simulink model "Demo_Shore"  (R2014a)
settings: Solver=FixedStepDiscrete  SolverMode=SingleTasking  StartTime=0.0  StopTime=inf  FixedStep=0.01  RelTol=1e-3
PostLoadFcn:
  | h_RPStest = RPStest;
model workspace (MAT data in the model file):
  gtest = 0
undefined symbols (not defined in the file or in its folder): avert, avert_gaze_dirs_chance, avert_gaze_duration_factor, avert_head_frequency_factor, avert_head_speed, BML, BML1, BML2, bmlsL, bmlsM, bodyBusyFlag, clock, emotion_amount_factor, faceBusyFlag, fileID, GAZE_WIN, gazing, mutual_gaze_duration_factor, P, pose_chanc_factor, pose_chance_factor, pose_change_flag, pose_frequency_factor, pose_lean, pose_lean_flag, pose_selfAdaptor_chance_factor, pose_speed, pr, serial, STATE_BEFORE, STATE_GO, STATE_OVER, STATE_READY, Stateflow
libraries: simulink x23, instrumentlib x6, lib_affectiveChar_behavior x3, realtime_pacer_lib x2, lib_affectiveChar_input x1
(part 2 of 7)

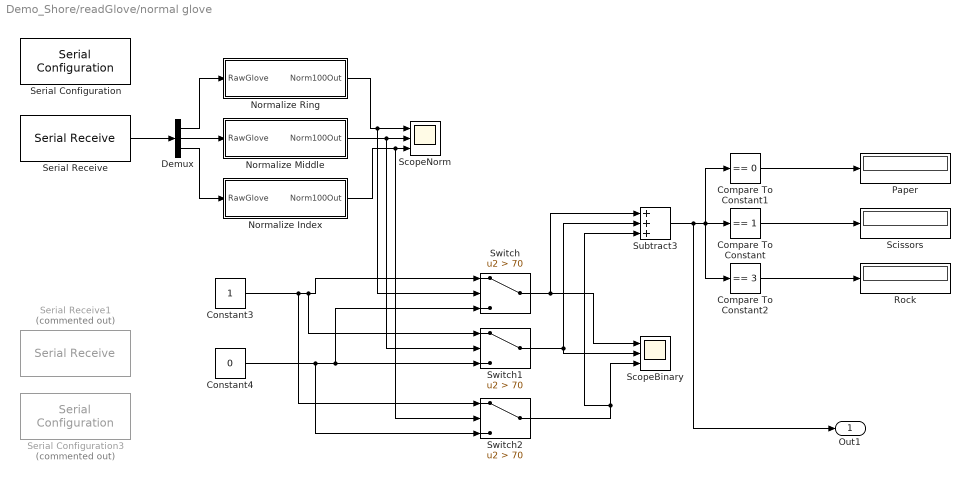
== system Demo_Shore/readGlove/normal glove ==
  Compare To Constant : simulink/Logic and Bit Operations/Compare To Constant  relop===  const=1  OutDataTypeStr=boolean
  Compare To Constant1 : simulink/Logic and Bit Operations/Compare To Constant  relop===  const=0  OutDataTypeStr=boolean
  Compare To Constant2 : simulink/Logic and Bit Operations/Compare To Constant  relop===  const=3  OutDataTypeStr=boolean
  Constant3 : Constant
  Constant4 : Constant  Value=0
  Demux : Demux  Outputs=3
  Normalize Index : Subsystem
  Normalize Middle : Subsystem
  Normalize Ring : Subsystem
  Paper : Display
  Rock : Display
  Scissors : Display
  ScopeBinary : Scope  NumInputPorts=3
      settings: YMin=-0.5~-0.5~-0.5  YMax=1.5~1.5~1.5
  ScopeNorm : Scope  NumInputPorts=3
      settings: TimeRange=10  YMin=-20~-20~-20  YMax=150~150~150
  Serial Configuration : instrumentlib/Serial Configuration  Priority=-200000  ComPortMenu=COM4  ComPort=COM4  ObjConstructor=serial('COM4');  BaudRate=9600  DataBits=8  Parity=none  StopBits=1  FlowControl=none  Timeout=10  ByteOrder=LittleEndian
  Serial Configuration3 : instrumentlib/Serial Configuration  Priority=-200000  Commented=on  ComPortMenu=<Please select a port...>  ComPort=COM5  ObjConstructor=serial('COM5');  BaudRate=9600  DataBits=8  Parity=none  StopBits=1  FlowControl=none  Timeout=10  ByteOrder=LittleEndian
  Serial Receive : instrumentlib/Serial Receive  ComPortMenu=COM4  ComPort=COM4  ObjConstructor=serial('COM4');  Terminator=<none>  DataSize="[3  1]"  DataType=uint8  EnableBlockingMode=on  ActionDataUnavailable=Output last received value  CustomValue=0  SampleTime=0.01
  Serial Receive1 : instrumentlib/Serial Receive  Commented=on  ComPortMenu=<Please select a port...>  ComPort=COM5  ObjConstructor=serial('COM5');  Terminator=<none>  DataSize="[3  1]"  DataType=uint8  EnableBlockingMode=on  ActionDataUnavailable=Output last received value  CustomValue=0  SampleTime=0.01
  Subtract3 : Sum  Inputs=+++
  Switch : Switch  Criteria=u2 > Threshold  Threshold=70
  Switch1 : Switch  Criteria=u2 > Threshold  Threshold=70
  Switch2 : Switch  Criteria=u2 > Threshold  Threshold=70
  Out1 : Outport
  wires:
  Demux/1 -> Normalize Ring/1(RawGlove)
  Demux/2 -> Normalize Middle/1(RawGlove)
  Demux/3 -> Normalize Index/1(RawGlove)
  Switch/1 -> ScopeBinary/1, Subtract3/1
  Constant3/1 -> Switch2/1, Switch1/1, Switch/1
  Constant4/1 -> Switch2/3, Switch1/3, Switch/3
  Switch1/1 -> ScopeBinary/2, Subtract3/2
  Switch2/1 -> Subtract3/3, ScopeBinary/3
  Subtract3/1 -> Compare To Constant/1, Compare To Constant2/1, Compare To Constant1/1, Out1/1
  Compare To Constant1/1 -> Paper/1
  Compare To Constant/1 -> Scissors/1
  Compare To Constant2/1 -> Rock/1
  Normalize Index/1(Norm100Out) -> Switch2/2, ScopeNorm/3
  Normalize Ring/1(Norm100Out) -> Switch/2, ScopeNorm/1
  Normalize Middle/1(Norm100Out) -> ScopeNorm/2, Switch1/2
  Serial Receive/1 -> Demux/1

== system Demo_Shore/readSHORE/smile ==
  In1 : Inport
  ifSmile : MATLAB Function  TreatAsAtomicUnit=on
  Out1 : Outport
  wires:
  ifSmile/1(y) -> Out1/1
  In1/1 -> ifSmile/1(u)

== system Demo_Shore/GazeFollowSubsystem/reactiveGaze/createGazePawn/sendBML ==
  In1 : Inport  OutDataTypeStr=double  PortDimensions=[1000 1]
  f : TriggerPort  TriggerType=function-call
      settings: CopyFcn=Stateflow.SLINSF.SimulinkMan.removeBlockPreDeleteFcn  PreDeleteFcn=Stateflow.SLINSF.SimulinkMan.unsafePredeleteFcn
  C++ S-Function2 : S-Function  FunctionName=yarpSendText_sfun  Parameters='/sim/out/bml8', '/SB/in/bml'  EnableBusSupport=off
  wires:
  In1/1 -> C++ S-Function2/1

== system Demo_Shore/GazeFollowSubsystem/reactiveGaze/createGazePawn/sendSBM ==
  In2 : Inport  OutDataTypeStr=double  PortDimensions=[1000 1]
  f : TriggerPort  TriggerType=function-call
      settings: CopyFcn=Stateflow.SLINSF.SimulinkMan.removeBlockPreDeleteFcn  PreDeleteFcn=Stateflow.SLINSF.SimulinkMan.unsafePredeleteFcn
  C++ S-Function2 : S-Function  FunctionName=yarpSendText_sfun  Parameters='/sim/out/smb5', '/SB/in/sbm'  EnableBusSupport=off
  wires:
  In2/1 -> C++ S-Function2/1

== stateflow chart Demo_Shore/CharacterControl/RPS_Scenario ==
  note: avert=1 to gazeCamera first time.
  state stateGame [parallel]
    settings: executionOrder=1
    state stateSt1
      entry: STATE_READY=7;STATE_GO=1;STATE_HAND=2;STATE_OVER=3; STATE_BEFORE=4;
      STATE_RESULT=5;STATE_WAIT=6; gameState=STATE_READY;
      BORED=1;SAD=2;FRUST=3;FEAR=4;CONTEMPT=5;IDLE=6;HAPPY=7;EXCITE=8;
      round=0;avert=0;gazing=0; uHand=1; bHand=1; randSmile=0; userHand=3;bradHand=3;
      win=0; uWinT=0; bWinT=0; BOREDOM_THRESHOLD=10; boredom=0;t=1;
    state stateStart
      entry:
      randPoseChance=0;randAvertGazeChance=0;
      GAZE_GUI=1;GAZE_SOFTEYE=2;GAZE_USER_HAND=3;GAZE_WIN=4; P=0;
      [P,BML]=initialPoseTable(4);avert=1;avertH=1;
      n=encStr2Arr(' ');newBmlsH=[n n n n n];
      newBmlsH=insertQueue(bmlsH,BML2); bmlsH=newBmlsH;
    state saccadeFinish
      entry:  [P,BML2]=initialPoseTable(1);
      newBmlsH=insertQueue(bmlsH,BML2);
      bmlsH=newBmlsH;
    state gameOver
      entry:
      gameState=STATE_OVER;
      boredom=boredom-1;
      gazing=0;
    state checkGameOver
    state stateInit
      entry: gameState= STATE_READY;
    state gazeCamera
      entry:  [P,BML2]=initialPoseTable(2);avert=0;
      newBmlsH=insertQueue(bmlsH,BML2);
      bmlsH=newBmlsH;
    state stateReady
      entry:
      round=round+1;
      bradHand=3;
      userHand=3;
      win=0;gazing=0;
    state statePoseReady
    state stateGo
      entry:
      gameState= STATE_GO;
    state stateReadUserHand
      entry:uHand=inputUser;gazing=GAZE_USER_HAND;
      gameState=STATE_HAND;
    state stateShowHands
      entry:
      bradHand=bHand;
      userHand=uHand;
    state stateCompare
      entry: temp=uHand-bHand;
      diff=temp- 3.*floor(temp/3);gazing=0;
      gameState= STATE_RESULT;
    state stateUserWin
      entry:
      win=1;disp('userWon')
      uWinT=uWinT+1;
    state stateBradWin
      entry:
      win=2;disp('bradWon')
      bWinT=bWinT+1;
    state stateNoWin
      entry:disp('noneWon')
      win=0;
    state stateShowResult
      entry: gazing=GAZE_GUI;
      gameState= STATE_WAIT;
    (default) -> stateSt1
    stateSt1 -> stateStart
    stateStart -> saccadeFinish : after(t,secs)
    saccadeFinish -> checkGameOver
    checkGameOver -> gameOver [order 1] : [round==10]
    checkGameOver -> stateGame.stateInit [order 2] : after(t,secs)
    stateGame.stateInit -> gazeCamera : after(2*t,secs)
    (junction 4) -> checkGameOver : after(4*t,secs)
    gazeCamera -> stateReady : after(1,secs)
    stateReady -> stateReady [order 2] : [uHand==3]
    stateReady -> statePoseReady [order 1] : [boredom<BOREDOM_THRESHOLD-4]{boredom=boredom+1;}
    stateReady -> statePoseReady [order 3]
    statePoseReady -> stateGo : after(t,secs){ bHand=randArray(:,15);}
    stateGo -> stateReadUserHand : after(2*t,secs)
    stateReadUserHand -> stateReadUserHand [order 1] : [uHand==3]
    stateReadUserHand -> stateShowHands [order 2]
    stateShowHands -> stateCompare
    stateCompare -> stateUserWin [order 2] : [diff==2]
    stateCompare -> stateBradWin [order 1] : [diff==1]
    stateCompare -> stateNoWin [order 3] : [diff~=1 && diff~=2]
    stateNoWin -> (junction 160)
    stateUserWin -> (junction 160)
    stateBradWin -> (junction 160)
    (junction 160) -> stateShowResult
    stateShowResult -> (junction 4)
  state statePlayHand [parallel]
    settings: executionOrder=2
    state stateRandomeHand
    state wait
    state statePoseRock
      entry: r=3;
      [P,BML2]= rockPoseTable(r) ;
      newBmlsH=insertQueue(bmlsH,BML2);
      bmlsH=newBmlsH;
    state statePosePaper
      entry: pa=3;
      [P,BML2]=  paperPoseBradTable(pa);
      newBmlsH=insertQueue(bmlsH,BML2);
      bmlsH=newBmlsH;
    state statePoseScissors
      entry: s=3;
      [P,BML2]= scissorsPoseBradTable(s);
      newBmlsH=insertQueue(bmlsH,BML2);
      bmlsH=newBmlsH;
    (default) -> stateRandomeHand
    stateRandomeHand -> wait : [gameState==STATE_GO]
    (junction 47) -> stateRandomeHand
    wait -> (junction 45)
    (junction 45) -> (junction 44) [order 3] : [bHand==0]
    (junction 45) -> (junction 46) [order 2] : [bHand==2]
    (junction 44) -> statePoseScissors
    (junction 45) -> statePosePaper [order 1] : [bHand==1]
    (junction 46) -> statePoseRock
    statePoseRock -> (junction 47) : after(2*t,secs)
    statePosePaper -> (junction 47) : after(2*t,secs)
    statePoseScissors -> (junction 47) : after(2*t,secs)
  state stateGameOver [parallel]
    settings: executionOrder=3
    state stateInit
    state stateAgentNotWin
      entry:[P,BML]= idlePoseBradTable(randArray(:,16));
      newBmlsL=insertQueueLow(bmlsL,BML);
      bmlsL=newBmlsL;
    state stateAgentWin
      entry:  gazing=GAZE_WIN;
    state stateBoredom
    (default) -> stateGameOver.stateInit
    stateGameOver.stateInit -> (junction 66) : [gameState==STATE_OVER]
    (junction 66) -> stateAgentWin [order 2] : [uWinT<bWinT]
    (junction 66) -> stateAgentNotWin [order 1] : [uWinT>=bWinT]
    stateAgentNotWin -> stateBoredom
    stateAgentWin -> stateBoredom
    stateBoredom -> stateBoredom : after(5*t,secs)[boredom<BOREDOM_THRESHOLD-2]{boredom=boredom+1;}
  note: GUI is updated by bHand when
      | gameState changes to GO.
  state sendSBM(arg) [function]
  data: bmls function_input double size=[1000,5]; mBML function_input double size=[1000,1]; newBmls function_output double size=[1000,5]; bmls function_input double size=[1000,5]; myBML function_input double size=[1000,1]; newBmls function_output double size=[1000,5]; arg function_input double size=[256 1]; p function_output double size=1; bmlID function_input double; poseBML function_output double size=[1000,1]; p function_output double size=1; bmlID function_input double; poseBML function_output double size=[1000,1]; p function_output double size=1; bmlID function_input double; poseBML function_output double size=[1000,1]; sbmID function_input double; poseSBM function_output double size=[1000,1]; p function_output double size=1; bmlID function_input double; poseBML function_output double size=[1000,1]; p function_output double size=1; bmlID function_input double; poseBML function_output double size=[1000,1]; gameState output double size=1; inputUser input double size=1; bradHand output double size=1; userHand output double size=1; win output double size=1; temp data_store_memory size=1; diff data_store_memory size=1; uHand data_store_memory size=1; bHand data_store_memory size=1; bWinT output double size=1; uWinT output double size=1; randSmile data_store_memory size=1; boredom data_store_memory size=1; BOREDOM_THRESHOLD data_store_memory size=1; randAvertGazeChance data_store_memory size=1; randPoseChance data_store_memory size=1; r data_store_memory size=1; pa data_store_memory size=1; s data_store_memory size=1; P data_store_memory size=1 =0; avert data_store_memory size=1; GAZE_GUI data_store_memory size=1; GAZE_SOFTEYE data_store_memory size=1; GAZE_USER_HAND data_store_memory size=1; STATE_READY data_store_memory size=1 =0; STATE_GO data_store_memory size=1 =1; STATE_HAND data_store_memory size=1 =2; STATE_OVER data_store_memory size=1 =3; gazing data_store_memory size=1; GAZE_WIN data_store_memory size=1; STATE_BEFORE data_store_memory size=1 =4; STATE_RESULT data_store_memory size=1 =5; STATE_WAIT data_store_memory size=1 =6; HAPPY data_store_memory size=1 =4; SAD data_store_memory size=1 =4; CONTEMPT data_store_memory size=1 =4; BORED data_store_memory size=1 =4; FRUST data_store_memory size=1 =4; FEAR data_store_memory size=1 =4; IDLE data_store_memory size=1 =4; EXCITE data_store_memory size=1 =4; BML data_store_memory size=[256,1]; pr data_store_memory size=1; round output double size=1; fileID data_store_memory size=1; BML2 data_store_memory size=[256,1]; t data_store_memory size=1 =0; bmlsH data_store_memory size=1 =0; newBmlsH local double size=[1000,5]; n data_store_memory; bmlsL data_store_memory size=1 =0; newBmlsL local double size=[1000,5]; randArray input double size=[1,25]; personality input double size=1; avertH data_store_memory size=1
  events: secs input RISING_EDGE_EVENT
  function newBmls =insertQueue(bmls,mBML):
    | function newBmls =insertQueue(bmls,mBML)
    |     full=1;
    |     tempp=encStr2Arr(' ');
    |     newBmls=[tempp tempp tempp tempp tempp];
    |     for i = 1:5
    |         if (isequal(bmls(:,i),tempp))
    |             %add to end of the queue where its empty
    |             bmls(:,i)=mBML;
    |             full=0;
    |             break
    |         end
    |     end
    |     if(full~=0)
    |             %if queue full, shift all elements to left which removes the first one, then add to end
    |             bmls(:,1)= bmls(:,2);
    |             bmls(:,2)= bmls(:,3);
    |             bmls(:,3)= bmls(:,4);
    |             bmls(:,5)=mBML;
    |     end
    |     newBmls=bmls;
  function newBmls =insertQueueLow(bmls,myBML):
    | function newBmls =insertQueueLow(bmls,myBML)
    |     full=1;
    |     tempp=encStr2Arr(' ');
    |     newBmls=[tempp tempp tempp tempp tempp];
    |     for i = 1:5
    |         if (isequal(bmls(:,i),tempp))
    |             %add to end of the queue where its empty
    |             bmls(:,i)=myBML;
    |             full=0;
    |             break
    |         end
    |     end
    |     if(full~=0)
    |             %if queue full, shift all elements to left which removes the first one, then add to end
    |             bmls(:,1)= bmls(:,2);
    |             bmls(:,2)= bmls(:,3);
    |             bmls(:,3)= bmls(:,4);
    |             bmls(:,5)=myBML;
    | 
    |     end
    |     newBmls=bmls;
  function [p,poseBML] = rockPoseTable(bmlID):
    | function [p,poseBML] = rockPoseTable(bmlID)
    | 
    | aVarTruthTableCondition_1 = false;
    | aVarTruthTableCondition_2 = false;
    | aVarTruthTableCondition_3 = false;
    | 
    | 
    | % rock
    | 
    | aVarTruthTableCondition_1 = logical(bmlID==1);
    | 
    | % rock
    | 
    | aVarTruthTableCondition_2 = logical(bmlID==2);
    | 
    | % rockB
    | 
    | aVarTruthTableCondition_3 = logical(bmlID==3);
    | 
    | if (aVarTruthTableCondition_1)
    |     aFcnTruthTableAction_1();
    | elseif (aVarTruthTableCondition_2)
    |     aFcnTruthTableAction_2();
    | elseif (aVarTruthTableCondition_3)
    |     aFcnTruthTableAction_4();
    | else % Default
    |     aFcnTruthTableAction_1();
    | end
    | 
    | function aFcnTruthTableAction_1()
    | 
    | % rock
    | 
    | poseBML=encStr2Arr('<?xml version="1.0" ?><act><bml><animation name="ChrBrad@Idle01_BeatFistMidLf02" start="0" ready="1" stroke="2" relax="3" end="4" /></bml></act>'); p=2;
    | 
    | function aFcnTruthTableAction_2()
    | 
    | % rock2
    | 
    | poseBML=encStr2Arr('<?xml version="1.0" ?><act><bml><animation name="ChrBrad@Idle01_BeatFistMidLf01" start="0" ready="1" stroke="2" relax="3" end="4" /></bml></act>'); p=2;
    | 
    | function aFcnTruthTableAction_3()
    | 
    | % rock
    | 
    | poseBML=encStr2Arr('<?xml version="1.0" ?><act><bml><animation name="../data/ChrBrad/test_Shake_Fist.skm"/></bml></act>'); p=2;
    | 
    | function aFcnTruthTableAction_4()
    | 
    | % prep
    | 
    | poseBML=encStr2Arr('<?xml version="1.0" ?><act><bml><animation name="../data/ChrBrad/test_RPS_Prep.skm"/></bml></act>'); p=2;
  function [p,poseBML] = paperPoseBradTable(bmlID):
    | function [p,poseBML] = paperPoseBradTable(bmlID)
    | 
    | aVarTruthTableCondition_1 = false;
    | aVarTruthTableCondition_2 = false;
    | aVarTruthTableCondition_3 = false;
    | 
    | 
    | % paper
    | 
    | aVarTruthTableCondition_1 = logical(bmlID==1);
    | 
    | % paper2
    | 
    | aVarTruthTableCondition_2 = logical(bmlID==2);
    | 
    | % paperB
    | 
    | aVarTruthTableCondition_3 = logical(bmlID==3);
    | 
    | if (aVarTruthTableCondition_1)
    |     aFcnTruthTableAction_1();
    | elseif (aVarTruthTableCondition_2)
    |     aFcnTruthTableAction_2();
    | elseif (aVarTruthTableCondition_3)
    |     aFcnTruthTableAction_3();
    | else % Default
    |     aFcnTruthTableAction_3();
    | end
    | 
    | function aFcnTruthTableAction_1()
    | 
    | % paper
    | 
    | poseBML=encStr2Arr('<?xml version="1.0" ?><act><bml><animation name="ChrBrad@Idle01_OfferLf01" start="0" stroke="2" relax="3" end="4"/></bml></act>');p=2;
    | 
    | function aFcnTruthTableAction_2()
    | 
    | % paper2
    | 
    | poseBML=encStr2Arr('<?xml version="1.0" ?><act><bml><animation name="ChrBrad@Idle01_YouLf01" start="0" stroke="2" relax="3" end="4"/></bml></act>');p=2;
    | 
    | function aFcnTruthTableAction_3()
    | 
    | % paperBilly
    | 
    | poseBML=encStr2Arr('<?xml version="1.0" ?><act><bml><animation name="../data/ChrBrad/test_Use_Paper.skm" /></bml></act>');p=2;
  function [p,poseBML] = scissorsPoseBradTable(bmlID):
    | function [p,poseBML] = scissorsPoseBradTable(bmlID)
    | 
    | aVarTruthTableCondition_1 = false;
    | aVarTruthTableCondition_2 = false;
    | aVarTruthTableCondition_3 = false;
    | 
    | 
    | % scissors
    | 
    | aVarTruthTableCondition_1 = logical(bmlID==1);
    | 
    | % scissors2
    | 
    | aVarTruthTableCondition_2 = logical(bmlID==2);
    | 
    | % scissorsB
    | 
    | aVarTruthTableCondition_3 = logical(bmlID==3);
    | 
    | if (aVarTruthTableCondition_1)
    |     aFcnTruthTableAction_1();
    | elseif (aVarTruthTableCondition_2)
    |     aFcnTruthTableAction_3();
    | elseif (aVarTruthTableCondition_3)
    |     aFcnTruthTableAction_3();
    | else % Default
    |     aFcnTruthTableAction_1();
    | end
    | 
    | function aFcnTruthTableAction_1()
    | 
    | % scissors
    | 
    | poseBML=encStr2Arr('<?xml version="1.0" ?><act><bml><animation name="ChrBrad@Idle01_YouLf01"/></bml></act>');p=2;
    | 
    | function aFcnTruthTableAction_2()
    | 
    | % scissors2
    | 
    | poseBML=encStr2Arr('<?xml version="1.0" ?><act><bml><animation name="ChrBrad@Idle01_OfferLf01"/></bml></act>');p=2;
    | 
    | function aFcnTruthTableAction_3()
    | 
    | % scissorsBilly
    | 
    | poseBML=encStr2Arr('<?xml version="1.0" ?><act><bml><animation name="../data/ChrBrad/test_Use_Scissors.skm" /></bml></act>');p=2;
  function poseSBM = handPoseSBTable(sbmID):
    | function poseSBM = handPoseSBTable(sbmID)
    | 
    | aVarTruthTableCondition_1 = false;
    | aVarTruthTableCondition_2 = false;
    | aVarTruthTableCondition_3 = false;
    | aVarTruthTableCondition_4 = false;
    | 
    | 
    | % fingersClose
    | 
    | aVarTruthTableCondition_1 = logical(sbmID==1);
    | 
    | % fingersNeutral
    | 
    | aVarTruthTableCondition_2 = logical(sbmID==2);
    | 
    | % lshoulkderForward
    | 
    | aVarTruthTableCondition_3 = logical(sbmID==3);
    | 
    | % lshoulkderNeutral
    | 
    | aVarTruthTableCondition_4 = logical(sbmID==4);
    | 
    | if (aVarTruthTableCondition_1)
    |     aFcnTruthTableAction_1();
    | elseif (aVarTruthTableCondition_2)
    |     aFcnTruthTableAction_2();
    | elseif (aVarTruthTableCondition_3)
    |     aFcnTruthTableAction_3();
    | elseif (aVarTruthTableCondition_4)
    |     aFcnTruthTableAction_4();
    | else % Default
    |     aFcnTruthTableAction_1();
    | end
    | 
    | function aFcnTruthTableAction_1()
    | 
    | % fingersClose
    | 
    | poseSBM=encStr2Arr('brad.getSkeleton().getJointByName("l_pinky1").setPostrotation(SrQuat(1,0,0,0.5));brad.getSkeleton().getJointByName("l_ring1").setPostrotation(SrQuat(1,0,0,0.5))');
    | 
    | function aFcnTruthTableAction_2()
    | 
    | % fingersNeutral
    | 
    | poseSBM=encStr2Arr('brad.getSkeleton().getJointByName("l_pinky1").setPostrotation(SrQuat(1,0,0,0));brad.getSkeleton().getJointByName("l_ring1").setPostrotation(SrQuat(1,0,0,0))');
    | 
    | function aFcnTruthTableAction_3()
    | 
    | % lshoulkderForward
    | 
    | poseSBM=encStr2Arr('brad.getSkeleton().getJointByName("l_sternoclavicular").setPostrotation(SrQuat(1,0,0,0.05))');
    | 
    | function aFcnTruthTableAction_4()
    | 
    | % lshoulkderNeutral
    | 
    | poseSBM=encStr2Arr('brad.getSkeleton().getJointByName("l_sternoclavicular").setPostrotation(SrQuat(1,0,0,0))');
  function [p,poseBML]=idlePoseBradTable(bmlID):
    | function [p,poseBML]=idlePoseBradTable(bmlID)
    | 
    | aVarTruthTableCondition_1 = false;
    | aVarTruthTableCondition_2 = false;
    | aVarTruthTableCondition_3 = false;
    | aVarTruthTableCondition_4 = false;
    | aVarTruthTableCondition_5 = false;
    | aVarTruthTableCondition_6 = false;
    | aVarTruthTableCondition_7 = false;
    | aVarTruthTableCondition_8 = false;
    | aVarTruthTableCondition_9 = false;
    | aVarTruthTableCondition_10 = false;
    | aVarTruthTableCondition_11 = false;
    | aVarTruthTableCondition_12 = false;
    | aVarTruthTableCondition_13 = false;
    | aVarTruthTableCondition_14 = false;
    | aVarTruthTableCondition_15 = false;
    | aVarTruthTableCondition_16 = false;
    | aVarTruthTableCondition_17 = false;
    | aVarTruthTableCondition_18 = false;
    | 
    | 
    | 
    | aVarTruthTableCondition_1 = logical(bmlID==1);
    | 
    | 
    | aVarTruthTableCondition_2 = logical(bmlID==2);
    | 
    | 
    | aVarTruthTableCondition_3 = logical(bmlID==3);
    | 
    | 
    | aVarTruthTableCondition_4 = logical(bmlID==4);
    | 
    | 
    | aVarTruthTableCondition_5 = logical(bmlID==5);
    | 
    | 
    | aVarTruthTableCondition_6 = logical(bmlID==6);
    | 
    | 
    | aVarTruthTableCondition_7 = logical(bmlID==7);
    | 
    | 
    | aVarTruthTableCondition_8 = logical(bmlID==8);
    | 
    | 
    | aVarTruthTableCondition_9 = logical(bmlID==9);
    | 
    | 
    | aVarTruthTableCondition_10 = logical(bmlID==10);
    | 
    | 
    | aVarTruthTableCondition_11 = logical(bmlID==11);
    | 
    | 
    | aVarTruthTableCondition_12 = logical(bmlID==12);
    | 
    | 
    | aVarTruthTableCondition_13 = logical(bmlID==13);
    | 
    | 
    | aVarTruthTableCondition_14 = logical(bmlID==14);
    | 
    | 
    | aVarTruthTableCondition_15 = logical(bmlID==15);
    | 
    | 
    | aVarTruthTableCondition_16 = logical(bmlID==16);
    | 
    | 
    | aVarTruthTableCondition_17 = logical(bmlID==17);
    | 
    | 
    | aVarTruthTableCondition_18 = logical(bmlID==18);
    | 
    | if (aVarTruthTableCondition_1)
    |     aFcnTruthTableAction_1();
    | elseif (aVarTruthTableCondition_2)
    |     aFcnTruthTableAction_2();
    | elseif (aVarTruthTableCondition_3)
    |     aFcnTruthTableAction_3();
    | elseif (aVarTruthTableCondition_4)
    |     aFcnTruthTableAction_4();
    | elseif (aVarTruthTableCondition_5)
    |     aFcnTruthTableAction_5();
    | elseif (aVarTruthTableCondition_6)
    |     aFcnTruthTableAction_11();
    | elseif (aVarTruthTableCondition_7)
    |     aFcnTruthTableAction_3();
    | elseif (aVarTruthTableCondition_8)
    |     aFcnTruthTableAction_5();
    | elseif (aVarTruthTableCondition_9)
    |     aFcnTruthTableAction_3();
    | elseif (aVarTruthTableCondition_10)
    |     aFcnTruthTableAction_10();
    | elseif (aVarTruthTableCondition_11)
    |     aFcnTruthTableAction_11();
    | elseif (aVarTruthTableCondition_12)
    |     aFcnTruthTableAction_8();
    | elseif (aVarTruthTableCondition_13)
    |     aFcnTruthTableAction_8();
    | elseif (aVarTruthTableCondition_14)
    |     aFcnTruthTableAction_7();
    | elseif (aVarTruthTableCondition_15)
    |     aFcnTruthTableAction_6();
    | elseif (aVarTruthTableCondition_16)
    |     aFcnTruthTableAction_5();
    | elseif (aVarTruthTableCondition_17)
    |     aFcnTruthTableAction_8();
    | elseif (aVarTruthTableCondition_18)
    |     aFcnTruthTableAction_9();
    | else % Default
    |     aFcnTruthTableAction_3();
    | end
    | 
    | function aFcnTruthTableAction_1()
    | 
    | % ArmStretchHandsFW
    | 
    | poseBML=encStr2Arr('<?xml version="1.0" ?><act><bml><animation name="ChrBrad@Idle01_ArmStretch01"/></bml></act>');p=3;
    | 
    | function aFcnTruthTableAction_2()
    | 
    | % HandsOnWaist
    | 
    | poseBML=encStr2Arr('<?xml version="1.0" ?><act><bml><animation name="ChrBrad@Idle01_ToIdle03"/></bml></act>');p=3;
    | 
    | function aFcnTruthTableAction_3()
    | 
    | % WeightShift
    | 
    | poseBML=encStr2Arr('<?xml version="1.0" ?><act><bml><animation name="ChrBrad@Idle01_WeightShift01" /></bml></act>');p=3;
    | 
    | function aFcnTruthTableAction_4()
    | 
    | % ScratchChest
    | 
    | poseBML=encStr2Arr('<?xml version="1.0" ?><act><bml><animation name="ChrBrad@Idle01_ScratchChest01" /></bml></act>');p=3;
    | 
    | function aFcnTruthTableAction_5()
    | 
    | % ScratchHead
    | 
    | poseBML=encStr2Arr('<?xml version="1.0" ?><act><bml><animation name="ChrBrad@Idle01_ScratchHeadLf01" /></bml></act>');p=3;
    | 
    | function aFcnTruthTableAction_6()
    | 
    | % ShoulderStretchUpDown
    | 
    | poseBML=encStr2Arr('<?xml version="1.0" ?><act><bml><animation name="ChrBrad@Idle01_ShoulderStretch01" /></bml></act>');p=3;
    | 
    | function aFcnTruthTableAction_7()
    | 
    | % scratchtemple(head)
    | 
    | poseBML=encStr2Arr('<?xml version="1.0" ?><act><bml><animation name="ChrBrad@Idle01_ScratchTempleLf01" /></bml></act>');p=3;
    | 
    | function aFcnTruthTableAction_8()
    | 
    | % SqueezeHand01
    | 
    | poseBML=encStr2Arr('<?xml version="1.0" ?><act><bml><animation name="ChrBrad@Idle01_SqueezeHand01" /></bml></act>');p=3;
    | 
    | function aFcnTruthTableAction_9()
    | 
    | % TouchHands01
    | 
    | poseBML=encStr2Arr('<?xml version="1.0" ?><act><bml><animation name="ChrBrad@Idle01_TouchHands01" /></bml></act>');p=3;
    | 
    | function aFcnTruthTableAction_10()
    | 
    | % WeightShift2
    | 
    | poseBML=encStr2Arr('<?xml version="1.0" ?><act><bml><animation name="ChrBrad@Idle01_WeightShift02" /></bml></act>');p=3;
    | 
    | function aFcnTruthTableAction_11()
    | 
    | % Idle01_ToIdle02
    | 
    | poseBML=encStr2Arr('<?xml version="1.0" ?><act><bml><animation name="ChrBrad@Idle01_ToIdle02" /></bml></act>');p=3;
  function [p,poseBML]=initialPoseTable(bmlID):
    | function [p,poseBML]=initialPoseTable(bmlID)
    | 
    | aVarTruthTableCondition_1 = false;
    | aVarTruthTableCondition_2 = false;
    | aVarTruthTableCondition_3 = false;
    | aVarTruthTableCondition_4 = false;
    | 
    | 
    | 
    | aVarTruthTableCondition_1 = logical(bmlID==1);
    | 
    | 
    | aVarTruthTableCondition_2 = logical(bmlID==2);
    | 
    | 
    | aVarTruthTableCondition_3 = logical(bmlID==3);
    | 
    | 
    | aVarTruthTableCondition_4 = logical(bmlID==4);
    | 
    | if (aVarTruthTableCondition_1)
    |     aFcnTruthTableAction_1();
    | elseif (aVarTruthTableCondition_2)
    |     aFcnTruthTableAction_2();
    | elseif (aVarTruthTableCondition_3)
    |     aFcnTruthTableAction_3();
    | elseif (aVarTruthTableCondition_4)
    |     aFcnTruthTableAction_4();
    | else % Default
    |     aFcnTruthTableAction_1();
    | end
    | 
    | function aFcnTruthTableAction_1()
    | 
    | % saccadeFinish
    | 
    | poseBML=encStr2Arr('<?xml version="1.0" ?><act><bml><saccade finish="true"/></bml></act>');p=3;
    | 
    | function aFcnTruthTableAction_2()
    | 
    | % neutralHeadGaze
    | 
    | poseBML=encStr2Arr('<?xml version="1.0" ?><act><bml><gaze target="camera" sbm:time-hint="0.2"/></bml></act>');p=3;
    | 
    | function aFcnTruthTableAction_3()
    | 
    | % blink
    | 
    | poseBML=encStr2Arr('<?xml version="1.0" ?><act><bml><face type="FACS" side="BOTH" au="45" amount="0.5" /></bml></act>');p=3;
    | 
    | function aFcnTruthTableAction_4()
    | 
    | % walkToN
    | 
    | poseBML=encStr2Arr( '<?xml version="1.0" ?><act><bml><locomotion manner="walk" facing="camera"  sbm:accel="0.5" sbm:scootaccel="50" target="0 0"/></bml></act>');p=3;

== stateflow chart Demo_Shore/CharacterControl/attention_Controller ==
  state setBodyFlag [parallel]
    settings: executionOrder=1
    state wait
      entry: timer=20;
    state init
      entry: bodyBusyFlag=0;timer=1;
    state flagOne
      entry:  bodyBusyFlag=1;
    state check
    state flagZero
      entry: bodyBusyFlag=0;
    (default) -> init
    init -> check
    flagOne -> wait [order 1] : [body_isAttending==1]
    wait -> flagOne
    check -> flagOne : [body_isAttending==1]
    flagZero -> check
    flagOne -> flagZero [order 2] : after(timer,secs)
  state setFaceFlag [parallel]
    settings: executionOrder=2
    state wait2
      entry: timer2=10;
    state init2
      entry: faceBusyFlag=0;timer2=1;
    state flagOne2
      entry:  faceBusyFlag=1;
    state check2
    state flagZero2
      entry: faceBusyFlag=0;
    (default) -> init2
    init2 -> check2
    flagOne2 -> wait2 [order 1] : [face_isAttending==1]
    wait2 -> flagOne2
    check2 -> flagOne2 : [face_isAttending==1]
    flagZero2 -> check2
    flagOne2 -> flagZero2 [order 2] : after(timer2,secs)
  data: bodyBusyFlag data_store_memory size=1; body_isAttending input; timer local; face_isAttending input; faceBusyFlag data_store_memory size=1; timer2 local
  events: secs input RISING_EDGE_EVENT

== stateflow chart Demo_Shore/CharacterControl/facialExpression_Controller ==
  state subSmile [parallel]
    settings: executionOrder=1
    state stateInitial
      entry: avert=1; gameState=14;
      n=encStr2Arr(' ');bmlsM=[n n n n n];newBmlsM=[n n n n n];
    state stateCheckSmile
    state gazeCamera
      entry:  [P,BMLM]= smileTable(2) ;avert=0;
      newBmlsM=insertQueue(bmlsM,BMLM);
      bmlsM=newBmlsM;
    state wait
    state checkP
      entry:  [P,BMLM]=  smileTable(1) ;
      newBmlsM=insertQueue(bmlsM,BMLM);
      bmlsM=newBmlsM;
    (default) -> stateInitial
    stateInitial -> stateCheckSmile
    stateCheckSmile -> stateCheckSmile [order 2]
    gazeCamera -> stateCheckSmile [order 2] : after(1,secs)[isSmiling~=1]
    subSmile.wait -> stateCheckSmile : after(10,secs)
    stateCheckSmile -> gazeCamera [order 1] : [[isSmiling==1]&[ gameState~= STATE_GO]&[ gameState~= STATE_READY]]
    checkP -> subSmile.wait
    gazeCamera -> checkP [order 1] : after(1,secs)[isSmiling==1]
  note: SMILE_DUER=10 seceonds
  note: check if still isSmiling is true works as a buffer to remove the smiles that last ony 1 sec (system errors).
  state subFacial [parallel]
    settings: executionOrder=2
    state stateFacialExpression
      entry:[au,au_L]=setAU(internalE);
      emotion_amount_factor =set_eAmountFactor(internalE,personality,emotion_amount_custom)
      BMLl=cmdBML_AUmerg(au,emotion_amount_factor);
      newBmlsL=insertQueueLow(bmlsL,BMLl);
      bmlsL=newBmlsL;
      %fprintf('%1.1f',internalE);disp(decArr2Str(BMLl));
    state initial
      entry:
      au=[0,0,0,0,0,0];
      au_L=0;
    state wait
    state wait2
    (default) -> initial
    subFacial.wait -> stateFacialExpression [order 1] : [internalE~=6]
    initial -> subFacial.wait
    stateFacialExpression -> subFacial.wait [order 1] : [internalE==6]
    subFacial.wait -> subFacial.wait [order 2]
    wait2 -> stateFacialExpression : [emoChange==1]
    stateFacialExpression -> wait2 [order 2] : [emoChange==0]
  data: bmls function_input double size=[1000,5]; myBML function_input double size=[1000,1]; newBmls function_output double size=[1000,5]; bmls function_input double size=[1000,5]; myBML function_input double size=[1000,1]; newBmls function_output double size=[1000,5]; bmlID function_input double; p function_output double size=1; poseBML function_output double size=[1000,1]; bmlID function_input double; p function_output double size=1; poseBML function_output double size=[1000,1]; E function_input double size=1; AU function_output double size=[1,6]; L function_output double size=1; E function_input double size=1; eAmountFactor function_output double size=[1,6]; p function_input double size=1; cFactor function_input double size=1; smileN local double size=1; isSmiling input double size=1 =0; avert data_store_memory =0; gazing data_store_memory size=2; GAZE_WIN data_store_memory size=2; BML data_store_memory size=[256,1]; P data_store_memory; fileID local double size=1; gameState output double; STATE_GO data_store_memory; STATE_READY data_store_memory; STATE_BEFORE data_store_memory; newBmlsM local double size=[1000,5]; bmlsM data_store_memory size=[256,1]; BMLM local double size=[1000,1]; n local; personality input double size=1; internalE input double size=1; au local; emotion_amount_factor data_store_memory; emoChange input boolean size=1; au_i local double size=1; au_L local double size=1; emoDisp local; bmlsL data_store_memory size=[256,1]; BMLl local double size=[1000,1]; newBmlsL local double size=[1000,5]; emotion_amount_custom input double size=1
  events: secs input RISING_EDGE_EVENT
  function newBmls =insertQueue(bmls,myBML):
    | function newBmls =insertQueue(bmls,myBML)
    |     full=1;
    |     t=encStr2Arr(' ');
    |     newBmls=[t t t t t];
    |     for i = 1:5
    |         if (isequal(bmls(:,i),t))
    |             %add to end of the queue where its empty
    |             bmls(:,i)=myBML;
    |             full=0;
    |             break
    |         end
    |     end
    |     if(full~=0)
    |             %if queue full, shift all elements to left which removes the first one, then add to end
    |             bmls(:,1)= bmls(:,2);
    |             bmls(:,2)= bmls(:,3);
    |             bmls(:,3)= bmls(:,4);
    |             bmls(:,5)=myBML;
    |     end
    |     newBmls=bmls;
  function newBmls =insertQueueLow(bmls,myBML):
    | function newBmls =insertQueueLow(bmls,myBML)
    |     full=1;
    |     t=encStr2Arr(' ');
    |     newBmls=[t t t t t];
    |     for i = 1:5
    |         if (isequal(bmls(:,i),t))
    |             %add to end of the queue where its empty
    |             bmls(:,i)=myBML;
    |             full=0;
    |             break
    |         end
    |     end
    |     if(full~=0)
    |             %if queue full, shift all elements to left which removes the first one, then add to end
    |             bmls(:,1)= bmls(:,2);
    |             bmls(:,2)= bmls(:,3);
    |             bmls(:,3)= bmls(:,4);
    |             bmls(:,5)=myBML;
    |     end
    |     newBmls=bmls;
  function [p,poseBML] = smileTable(bmlID):
    | function [p,poseBML] = smileTable(bmlID)
    | 
    | aVarTruthTableCondition_1 = false;
    | aVarTruthTableCondition_2 = false;
    | 
    | 
    | % smile
    | 
    | aVarTruthTableCondition_1 = logical(bmlID==1);
    | 
    | % headN
    | 
    | aVarTruthTableCondition_2 = logical(bmlID==2);
    | 
    | if (aVarTruthTableCondition_1)
    |     aFcnTruthTableAction_1();
    | elseif (aVarTruthTableCondition_2)
    |     aFcnTruthTableAction_2();
    | else % Default
    |     aFcnTruthTableAction_1();
    | end
    | 
    | function aFcnTruthTableAction_1()
    | 
    | % smile
    | 
    | poseBML=encStr2Arr('<?xml version="1.0"?><act><bml><face amount="1" au="12" side="BOTH" start="0" stroke="2" relax="3" end="4" type="facs"/><face amount="0.3" au="6" side="BOTH" start="0" stroke="2" relax="3" end="4" type="facs"/></bml></act>');p=3;
    | 
    | function aFcnTruthTableAction_2()
    | 
    | % headNeutralBrow
    | 
    | poseBML=encStr2Arr('<?xml version="1.0" ?><act><bml><gaze target="gazeTarget" start="0" end="5" sbm:time-hint="1.5"/></bml></act>');p=3;
    | 
    | function aFcnTruthTableAction_3()
    | 
    | % smileBrow
    | 
    | poseBML=encStr2Arr('<?xml version="1.0"?><act><bml><face amount="0.1" au="1" side="BOTH" start="0" stroke="2" relax="4" end="6" type="facs"/><face amount="0.1" au="2" side="BOTH" start="0" stroke="2" relax="4" end="6" type="facs"/></bml></act>');p=3;
  function [p,poseBML] = facialExpr(bmlID):
    | function [p,poseBML] = facialExpr(bmlID)
    | 
    | aVarTruthTableCondition_1 = false;
    | aVarTruthTableCondition_2 = false;
    | 
    | 
    | % smile
    | 
    | aVarTruthTableCondition_1 = logical(bmlID==1);
    | 
    | % headN
    | 
    | aVarTruthTableCondition_2 = logical(bmlID==2);
    | 
    | if (aVarTruthTableCondition_1)
    |     aFcnTruthTableAction_1();
    | elseif (aVarTruthTableCondition_2)
    |     aFcnTruthTableAction_2();
    | else % Default
    |     aFcnTruthTableAction_1();
    | end
    | 
    | function aFcnTruthTableAction_1()
    | 
    | % smile
    | 
    | poseBML=encStr2Arr('<?xml version="1.0"?><act><bml><face amount="1" au="12" side="BOTH" start="0" stroke="10" relax="70" end="100" type="facs"/><face amount="0.3" au="6" side="BOTH" start="0" stroke="10" relax="70" end="100" type="facs"/></bml></act>');p=3;
    | 
    | function aFcnTruthTableAction_2()
    | 
    | % headNeutralBrow
    | 
    | poseBML=encStr2Arr('<?xml version="1.0" ?><act><bml><gaze target="gazeTarget" start="0" end="5" sbm:time-hint="1.5"/></bml></act>');p=3;
    | 
    | function aFcnTruthTableAction_3()
    | 
    | % smileBrow
    | 
    | poseBML=encStr2Arr('<?xml version="1.0"?><act><bml><face amount="0.1" au="1" side="BOTH" start="0" stroke="2" relax="4" end="6" type="facs"/><face amount="0.1" au="2" side="BOTH" start="0" stroke="2" relax="4" end="6" type="facs"/></bml></act>');p=3;
  function [AU,L]=setAU(E):
    | function [AU,L]=setAU(E)	
    | % 1	Inner Brow Raiser,% 2	Outer Brow Raiser, % 4	Brow Lowerer
    | % 5	Upper Lid Raiser,% 6	Cheek Raiser,% 7	Lid Tightener
    | % 8	Lips Toward Each Other,% 9	Nose Wrinkler,% 10	Upper Lip Raiser	
    | % 11	Nasolabial Deepener	% 12	Lip Corner Puller % 13	Sharp Lip Puller % 14	Dimpler	
    | % 15	Lip Corner Depressor % 16	Lower Lip Depressor % 17	Chin Raiser	mentalis
    | % 18	Lip Pucker	% 19	Tongue Show	% 20	Lip Stretcher % 21	Neck Tightener	platysma
    | % 22	Lip Funneler% 23	Lip Tightener% 24	Lip Pressor % 25	Lips Part	depressor
    | % 26	Jaw Drop,% 27	Mouth Stretch
    | % 43	Eyes Closed, % 44	Eyebrow Gatherer,% 45	Blink,% 46	Wink
    | %smartbody no 43,15,17,10 looks wierd,no 142
    |    AU=[0,0,0,0,0,0];L=0;
    |    % AU5(eyeOpen) for A+
    |    % AU1,4 for V-
    |    %AU12 for V+
    |     switch(E)
    |         case 1 %V- A-,bored (43)[1]
    |             AU=[1,2,45,0,0,0];L=3;%[1,1,0.35]
    |         
    |         case 2 %V- A-;sad %(1,2,4,10,15,17,43)[];can be [1,2,4,45,6,0]
    |             AU=[1,4,0,0,0,0];L=2;%[1,1,0,0,0,0]
    |         
    |         case 3 %V- A+,frust(2,1,14)[1],(-1,-2,4,7,14)[2], maybe(1,7)[0.7,0.7,0.5]
    |             AU=[1,2,4,5,6,0];L=5;%[1,1,1,0.5,0.5,0]
    |         
    |         case 4 %V- A+,fear(1,2,4,5,25=mouth)
    |             AU=[1,2,4,5,6,7];L=6; %[1,1,1,0.2,0.2]
    |         
    |         case 5%V+ A-,calm
    |             AU=[12,14,0,0,0,0];L=2;%[0.7,0.3,0,0,0,0]
    |         
    |         case 7%V+ A+,happy
    |             AU=[6,12,0,0,0,0];L=2;%[1,0.5,0,0,0,0]
    |         
    |         case 8%V+ A+,excited
    |             AU=[12,26,5,1,2,0];L=5;%[1,1,1,1,1,0]
    |         
    |         case 9%V- A+, angry
    |             AU=[2,4,5,7,45,0];L=5;%[0.5,1,0.2,0.2,0.2]
    |         
    |         otherwise
    |             %confusion (1,2,4,7)[1] %[1,1,1,0.2]
    |             %worried (1,2,4,5) [1,1,1,0.5]
    |             %angry(4,5,7,10,27)[], can be(2,4,5,7,45)[0.5,1,0.2,0.2,0.2]
    | 
    |             AU=[0,0,0,0,0,0];L=0;
    |             disp('error, setAU,emotion not listed');
    |     end  
    | %[1]Craig S.D. et al(2004)emotions during learning:the first steps tw affect sensitive
    | %[2]grafsgard J F () automatically recog facial indicator of frust
  function eAmountFactor =set_eAmountFactor(E,p,cFactor):
    | function eAmountFactor =set_eAmountFactor(E,p,cFactor)
    |     AU=[0,0,0,0,0,0];eAmountFactor=[0,0,0,0,0,0];pFactor=0.5;
    |     %Note: make sure you change values in all 4 personalities
    |     if(p==1)
    |         %HEHN
    |         if(E==1)  %bored
    |             eAmountFactor=[1,1,0.37,0,0,0];
    |         elseif(E==2) %sad
    |             eAmountFactor=[1,1,0,0,0,0];
    |         elseif(E==3) %frust
    |             eAmountFactor=[1,1,1,0.5,0.5,0];
    |         elseif(E==4) %fear
    |             eAmountFactor=[1,1,1,0.2,0.2,0];
    |         elseif(E==5)%sleepy
    |             eAmountFactor=[0.7,0.3,0,0,0,0];
    |         elseif(E==7)%happy
    |             eAmountFactor=[0.38,1,0,0,0,0];
    |         elseif(E==8)%excited
    |             eAmountFactor=[0.5,0.2,0.6,0.6,0.6,0];    
    |         else          
    |             eAmountFactor=[0,0,0,0,0,0];
    |             disp('error, set_eAmountFactor,emotion not listed');
    |         end
    |         eAmountFactor=eAmountFactor*cFactor;
    |         %LEHN  
    |     elseif(p==2)
    |         if(E==1)  %bored
    |             eAmountFactor=[1,1,0.37,0,0,0];
    |         elseif(E==2) %sad
    |             eAmountFactor=[1,1,0,0,0,0];
    |         elseif(E==3) %frust
    |             eAmountFactor=[1,1,1,0.5,0.5,0];
    |         elseif(E==4) %fear
    |             eAmountFactor=[1,1,1,0.2,0.2,0];
    |         elseif(E==5)%sleepy
    |             eAmountFactor=[0.7,0.3,0,0,0,0];
    |         elseif(E==7)%happy
    |             eAmountFactor=[0.38,1,0,0,0,0];
    |         elseif(E==8)%excited[12,26,5,1,2,0]
    |             eAmountFactor= [0.5,0.2,0.6,0.6,0.6,0];    
    |         else          
    |             eAmountFactor=[0,0,0,0,0,0];
    |             disp('error, set_eAmountFactor,emotion not listed');
    |         end
    |         eAmountFactor=eAmountFactor*cFactor;
    |         %HELN
    |    elseif(p==3)
    |         if(E==1)  %bored
    |             eAmountFactor=[1,1,0.37,0,0,0];
    |         elseif(E==2) %sad
    |             eAmountFactor=[1,1,0,0,0,0];
    |         elseif(E==3) %frust
    |             eAmountFactor=[1,1,1,0.5,0.5,0];
    |         elseif(E==4) %fear
    |             eAmountFactor=[1,1,1,0.2,0.2,0];
    |         elseif(E==5)%sleepy
    |             eAmountFactor=[0.7,0.3,0,0,0,0];
    |         elseif(E==7)%happy
    |             eAmountFactor=[0.38,1,0,0,0,0];
    |         elseif(E==8)%excited[12,26,5,1,2,0]
    |             eAmountFactor=  [0.5,0.2,0.6,0.6,0.6,0];    
    |         else          
    |             eAmountFactor=[0,0,0,0,0,0];
    |             disp('error, set_eAmountFactor,emotion not listed');
    |         end
    |         eAmountFactor=eAmountFactor*pFactor*cFactor;
    |         %LELN
    |     elseif(p==4)
    |         if(E==1)  %bored
    |             eAmountFactor=[1,1,0.37,0,0,0];
    |         elseif(E==2) %sad
    |             eAmountFactor=[1,1,0,0,0,0];
    |         elseif(E==3) %frust
    |             eAmountFactor=[1,1,1,0.5,0.5,0];
    |         elseif(E==4) %fear
    |             eAmountFactor=[1,1,1,0.2,0.2,0];
    |         elseif(E==5)%sleepy
    |             eAmountFactor=[0.7,0.3,0,0,0,0];
    |         elseif(E==7)%happy
    |             eAmountFactor=[0.38,1,0,0,0,0];
    |         elseif(E==8)%excited[12,26,5,1,2,0]
    |             eAmountFactor=  [0.5,0.2,0.6,0.6,0.6,0];    
    |         else          
    |             eAmountFactor=[0,0,0,0,0,0];
    |             disp('error, set_eAmountFactor,emotion not listed');
    |         end
    |         eAmountFactor=eAmountFactor*pFactor*cFactor;
    |     end
    | %Following is if we want a same factor for each personaliy all through AUs
    | % function eAmountFactor =set_eAmountFactor(E,P)
    | %     AU=[6,12,142,0,0,0];eAMOUNT=[0,0,0,0,0,0];
    | %     switch E
    | %         case 1  %bored
    | %             eAMOUNT=[1,1,1,0,0,0];
    | %         case 2 %sad
    | %             eAMOUNT=[0.7,0.4,0.9,0,0,0];
    | %         case 3 %angry
    | %             eAMOUNT=[1,0.8,1,0,0,0];
    | %         case 4 %fear
    | %             eAMOUNT=[1,1,1,0,0,0];%5,6,7,26
    | %         case 5%contempt
    | %             eAMOUNT=[1,1,1,0,0,0];
    | %         case 7%happy
    | %             eAMOUNT=[0.2,1,0,0,0,0];
    | %         otherwise           
    | %             eAMOUNT=[0,0,0,0,0,0];
    | %             disp('error,amount for emotion not listed:');disp('eAMOUNT');
    | %     end 
    | %     switch P
    | %         case 1 %HEHN
    | %             pFactor=1;
    | %         case 2 %LEHN
    | %             pFactor=1;
    | %         case 3 %HELN
    | %             pFactor=0.5;
    | %         case 4 %LELN
    | %             pFactor=0.5;
    | %     end
    | %     eAmountFactor=pFactor*eAMOUNT;

== matlab function Demo_Shore/EmotionSubsystem/calculateValenceArousal/HELN_VA_Emo ==
  data: V input; e output double size=1; A input double
function e = fcn(V, A)

aVarTruthTableCondition_1 = false;
aVarTruthTableCondition_2 = false;
aVarTruthTableCondition_3 = false;
aVarTruthTableCondition_4 = false;
aVarTruthTableCondition_5 = false;
aVarTruthTableCondition_6 = false;
aVarTruthTableCondition_7 = false;
aVarTruthTableCondition_8 = false;


% 7-happy  2,1

aVarTruthTableCondition_1 = logical(V>10 && A<10 && A>0);

% 8-ex  1,2 AND 2,2

aVarTruthTableCondition_2 = logical(V>0 && A>10);

% 4-fear  -1,2 AND -2,2

aVarTruthTableCondition_3 = logical(V<0 && A>10);

% 3-frust  -2,1

aVarTruthTableCondition_4 = logical(V<-10 && A<10 && A>0);

% 6-idle  2,-1

aVarTruthTableCondition_5 = logical(V>10 && A<0 && A>-10);

% 5-calm  1,-2 AND 2,-2

aVarTruthTableCondition_6 = logical(V>0 && A<-10);

% 1-bored  -1,-2 AND -2,-2

aVarTruthTableCondition_7 = logical(V<0 && A<-10);

% 2-sad  -2,-1

aVarTruthTableCondition_8 = logical(V<-10 && A<0 && A>-10);

if (aVarTruthTableCondition_1)
    aFcnTruthTableAction_1();
elseif (aVarTruthTableCondition_2)
    aFcnTruthTableAction_2();
elseif (aVarTruthTableCondition_3)
    aFcnTruthTableAction_3();
elseif (aVarTruthTableCondition_4)
    aFcnTruthTableAction_4();
elseif (aVarTruthTableCondition_5)
    aFcnTruthTableAction_5();
elseif (aVarTruthTableCondition_6)
    aFcnTruthTableAction_6();
elseif (aVarTruthTableCondition_7)
    aFcnTruthTableAction_7();
elseif (aVarTruthTableCondition_8)
    aFcnTruthTableAction_8();
else % Default
    aFcnTruthTableAction_5();
end

function aFcnTruthTableAction_1()

% happy

e=7;

function aFcnTruthTableAction_2()

% excited

e=8;

function aFcnTruthTableAction_3()

% fear

e=4;

function aFcnTruthTableAction_4()

% frustration

e=3;

function aFcnTruthTableAction_5()

% idle

e=6;

function aFcnTruthTableAction_6()

% contempt

e=5;

function aFcnTruthTableAction_7()

% bored

e=1;

function aFcnTruthTableAction_8()

% sad

e=2;

== matlab function Demo_Shore/EmotionSubsystem/satFunction ==
  data: randv input; smile input; wave input; win input; invade input; v_trig output; v_trigW output; vaFlag input
function [v_trig,v_trigW]= fcn(randv,smile,wave,win,invade,vaFlag)
%#codegen
%Maryam 30/06/2015
%Here set Agent's satisfaction flag based on your scenario

%In RPS scenario agent gets satisfined when she wins
    v_trig=0;%if 1 triggers V_A module to inserease valence
    v_trigW=1;%weight by which valence value is changed (sum of weight of all triggers)
if(vaFlag==1)
    % 30% chance of random increase or decrease in valence
    randTrigger=floor(randv);
    if(0<randTrigger)&&(randTrigger<30)
        v_trig=1;
        v_trigW=v_trigW+0.1;
    end
    if(30<randTrigger)&&(randTrigger<60)
        v_trig=-1;
        v_trigW=abs(v_trigW-0.1);
    end
    
    if(win==2) %agent wins so she is satisfied
        v_trig=1;
        v_trigW=v_trigW+0.5;
    elseif(win==1) %user wins so agent is NOT satisfied
        v_trig=-1;
        v_trigW=abs(v_trigW-0.5);
    end

    if(smile==1)
        v_trig=1;
        v_trigW=v_trigW+0.1;
    end

    if(wave==1)
        v_trig=1;
        v_trigW=v_trigW+0.1;
    end

    if(invade==1)
        v_trig=-1;
        v_trigW=abs(v_trigW-0.1);
    end
else
     v_trig=0;
     v_trigW=0;
end

== matlab function Demo_Shore/EmotionSubsystem/arousalFlagFunction ==
  data: userInvade input; interactionState input; randa input; a_trig output; a_trigW output; vaFlag input
function [a_trig,a_trigW]= fcn(userInvade,interactionState,randa,vaFlag)
%#codegen
%Maryam 30/06/2015
%Here set in which states of the interaction agent experienced 
% more arousal(arousalFlag=1) and less arousal (arousalFlag=-1)
%Note that you should define the states in your scenraio beforehand
%we assume agent gets more aroused when in ready/go state and 
%less aroused when in WAITE/HAND
if(vaFlag==1)
    a_trig=0; %if 1 triggers V_A module to inserease arousal
    a_trigW=1; %weight by which arousal value is changed (sum of weight of all triggers)
    
    % 30% chance of random increase or decrease in arousal
    randTrigger=floor(randa);
    if(0<randTrigger)&&(randTrigger<30)
        a_trig=1;
        a_trigW=a_trigW+0.1;
    end
    if(30<randTrigger)&&(randTrigger<60)
        a_trig=-1;
        a_trigW=abs(a_trigW - 0.1);
    end
    
    if(interactionState==1)%GO - highely aroused state
        a_trig=1;
        a_trigW=a_trigW+0.5;
    end
    if(interactionState==7)%READY - high aroused state
        a_trig= 1;
        a_trigW=a_trigW+0.5;
    end
    if(interactionState==2)%HAND- highely aroused state
        a_trig=-1;
        a_trigW=abs(a_trigW -0.5);
    end
    if(interactionState==6)%WAIT - low aroused state
        a_trig=-1;
        a_trigW=abs(a_trigW-0.5);
    end
    %     elseif(interactionState==3)%OVER - low aroused state
%         arousalTrig=-1;  
%         end
    if(userInvade==1)
       a_trig=1;
       a_trigW=a_trigW+0.1;
    end
else
    a_trig=0;
    a_trigW=0;
end

== stateflow chart Demo_Shore/GazeFollowSubsystem/reactiveGaze/createGazePawn ==
  state sendBML(In1) [function]
  state sendSBM(In2) [function]
  state stateCreatePawn
    entry:
    sendSBM( encStr2Arr( 'gt = scene.createPawn("gazeTarget")' ) );
    sendBML(encStr2Arr('<?xml version="1.0" ?><act><bml><gaze sbm:joint-range="EYES BACK" target="gazeTarget"/></bml></act>'));
  (default) -> stateCreatePawn
  data: In1 function_input double size=[1000 1]; In2 function_input double size=[1000 1]
